simulink model "Progetto_1b"  (R2020b)
settings: Solver=VariableStepAuto  StartTime=0.0  StopTime=2  MaxStep=1e-4  RelTol=1e-3
values from neighbouring files (symbols this model uses):
  A = [0 , 1 ... (first row only)    [1b.m]    (also in traccia_1b.m)
  B = [ 0 ... (first row only)    [1b.m]    (also in traccia_1b.m)
  C = [1 , 0]    [1b.m]    (also in traccia_1b.m)
  den_r = d_r{1}    [1b.m]    (also in traccia_1b.m)
  num_r = n_r{1}    [1b.m]    (also in traccia_1b.m)
  u_e = 3.8971    [1b.m]    (also in traccia_1b.m)
  W = -pi/3    (= -1.0471975512)    [1b.m]    (also in traccia_1b.m)
  w_n_min = 15 * 10^4    (= 150000)    [1b.m]    (also in traccia_1b.m)
  x0 = [0 0]    [1b.m]    (also in traccia_1b.m)
  x_e = [pi/3 0]    [1b.m]    (also in traccia_1b.m)
  ye = pi/3    (= 1.0471975512)    [1b.m]    (also in traccia_1b.m)
undefined symbols (not defined in the file or in its folder): Den, Num
settings Model: Creator=spiri  LastModifiedBy=franc

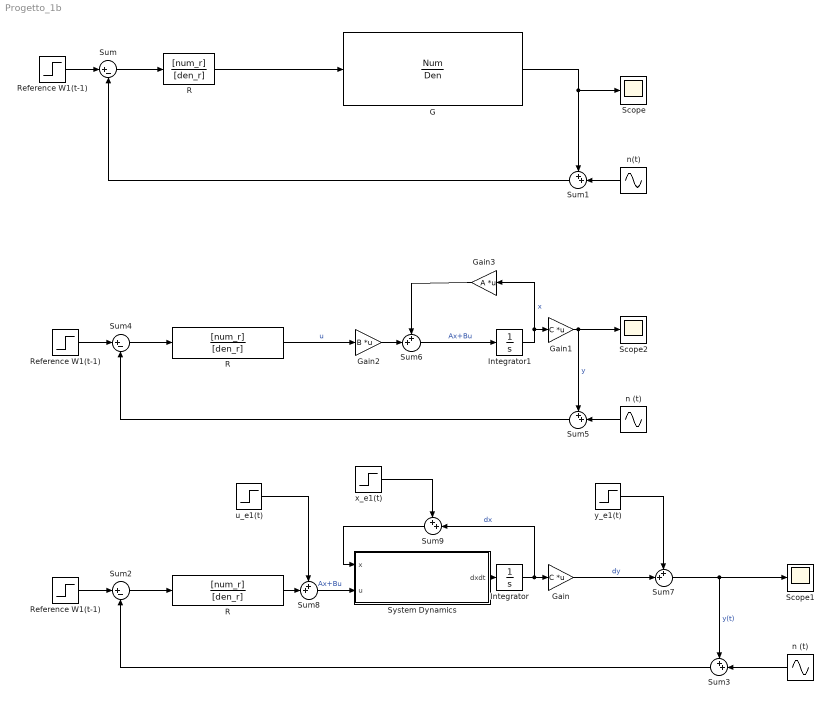
== system Progetto_1b ==
  G : TransferFcn  Numerator=Num  Denominator=Den
  Gain : Gain  Gain=C  Multiplication=Matrix(K*u)
  Gain1 : Gain  Gain=C  Multiplication=Matrix(K*u)
  Gain2 : Gain  Gain=B  Multiplication=Matrix(K*u)
  Gain3 : Gain  Gain=A  Multiplication=Matrix(K*u)
  Integrator : Integrator  InitialCondition=x_e
  Integrator1 : Integrator  InitialCondition=x0
  R : TransferFcn  Numerator=[num_r]  Denominator=[den_r]
  "R " : TransferFcn  Numerator=[num_r]  Denominator=[den_r]
  "R " : TransferFcn  Numerator=[num_r]  Denominator=[den_r]
  Reference W1(t-1) : Step  After=W  SampleTime=0
  "Reference W1(t-1) " : Step  After=W  SampleTime=0
  "Reference W1(t-1) " : Step  After=W  SampleTime=0
  Scope : Scope
  Scope1 : Scope
  Scope2 : Scope
  Sum : Sum  Inputs=|+-
  Sum{1,3,5..9} (7 alike) : Sum  Inputs=++|
  Sum2 : Sum  Inputs=|+-
  Sum4 : Sum  Inputs=|+-
  System Dynamics : MATLAB Function  TreatAsAtomicUnit=on
  n (t) : Sin  Amplitude=0.01  Frequency=w_n_min  SampleTime=0
  "n (t) " : Sin  Amplitude=0.01  Frequency=w_n_min  SampleTime=0
  n(t) : Sin  Amplitude=0.01  Frequency=w_n_min  SampleTime=0
  u_e1(t) : Step  Time=0  After=u_e  SampleTime=0
  x_e1(t) : Step  Time=0  After=x_e  SampleTime=0
  y_e1(t) : Step  Time=0  After=ye  SampleTime=0
  wires:
  n(t)/1 -> Sum1/2
  Sum1/1 -> Sum/2
  Reference W1(t-1)/1 -> Sum/1
  G/1 -> Scope/1, Sum1/1
  Sum/1 -> R/1
  R/1 -> G/1
  "R "/1 -> Sum8/2
  Sum2/1 -> "R "/1
  "Reference W1(t-1) "/1 -> Sum2/1
  Sum3/1 -> Sum2/2
  n (t)/1 -> Sum3/2
  System Dynamics/1(dxdt) -> Integrator/1
  Integrator/1 -> Sum9/2, Gain/1  "dx"
  Gain1/1 -> Sum5/1, Scope2/1  "y"
  Integrator1/1 -> Gain1/1, Gain3/1  "x"
  Sum6/1 -> Integrator1/1  "Ax+Bu"
  "n (t) "/1 -> Sum5/2
  Sum5/1 -> Sum4/2
  "Reference W1(t-1) "/1 -> Sum4/1
  Sum4/1 -> "R "/1
  "R "/1 -> Gain2/1  "u"
  Gain2/1 -> Sum6/2
  Gain3/1 -> Sum6/1
  Sum8/1 -> System Dynamics/2(u)  "Ax+Bu"
  u_e1(t)/1 -> Sum8/1
  Gain/1 -> Sum7/2  "dy"
  Sum7/1 -> Sum3/1, Scope1/1  "y(t)"
  y_e1(t)/1 -> Sum7/1
  x_e1(t)/1 -> Sum9/1
  Sum9/1 -> System Dynamics/1(x)

== matlab function Progetto_1b/System Dynamics ==
  data: x input; u input; dxdt output
function dxdt = systemDynamics(x,u)

%parametri delle equazioni;
beta=0.3; 
a=0.3; 
Id = 0.5;
Fv=-8.7;


dx1dt=x(2);
dx2dt= (-beta*x(2)+ (a/2)*sind(x(1))*Fv + a*u)/Id; 
%dxdt = [dx1dt; dx2dt; dx3dt;...;dxndt];
dxdt = [dx1dt; dx2dt;];
